simulink model "Furuta_pendulum"  (R2022b)
settings: Solver=ode45  StartTime=0.0  StopTime=3  MaxStep=0.1  RelTol=1e-3
values from neighbouring files (symbols this model uses):
  A = [ 0 0 1 0 ... (first row only)    [Initialize_parameters.m]    (also in Matlab_simulation.m)
  B = [ 0 0 ... (first row only)    [Initialize_parameters.m]    (also in Matlab_simulation.m)
  b1 = 0.01    [Initialize_parameters.m]    (also in Matlab_simulation.m)
  b1s = 0.00    (= 0)    [Initialize_parameters.m]    (also in Matlab_simulation.m = 0.001)
  b2 = 0.001    [Initialize_parameters.m]    (also in Matlab_simulation.m)
  C = ident    [Initialize_parameters.m]    (also in sysCLode.m = [ m2*l2^2*dth2*sin(th2)*cos(th2)+b1,          m2*l2^2*dth1*s)
  D = zeros(4,2)    [Initialize_parameters.m]
  epsilon = 1/sqrt(2)    [Initialize_parameters.m]
  g = 9.81    [Initialize_parameters.m]    (also in Matlab_simulation.m)
  ident = eye(4)    [Initialize_parameters.m]
  invC = inv(C)    [Initialize_parameters.m]
  J1 = 0.000027+0.00257    (= 0.002597)    [Initialize_parameters.m]    (also in Matlab_simulation.m)
  J2 = 4.15e-5    (= 4.15e-05)    [Initialize_parameters.m]    (also in Matlab_simulation.m)
  Ki = 2    [Initialize_parameters.m]
  Kt = 0.071    [Initialize_parameters.m]
  l1 = 0.16    [Initialize_parameters.m]    (also in Matlab_simulation.m)
  l2 = 0.075    [Initialize_parameters.m]    (also in Matlab_simulation.m)
  m2 = 0.0206    [Initialize_parameters.m]    (also in Matlab_simulation.m)
  tau2 = 0.00    (= 0)    [Initialize_parameters.m]    (also in sysCLode.m)
  Td = 0.01    [Initialize_parameters.m]
  tr = 3    [Initialize_parameters.m]
  ts_ZH = 0.001    [Initialize_parameters.m]
  Vmax = 3    [Initialize_parameters.m]
  x0 = [0; 5*deg2rad; 0; 0]    [Initialize_parameters.m]    (also in Matlab_simulation.m = [0; 5*pi/180; 0; 0])
  x_eq = [0; 0; 0; 0]    [Initialize_parameters.m]    (also in Matlab_simulation.m)
undefined symbols (not defined in the file or in its folder): Kinf
settings Model: Creator=lucaschenato  LastModifiedBy=luca.salviato
settings SolverCC: AlgebraicLoopSolver=TrustRegion
settings DataIOCC: ReturnWorkspaceOutputs=off
settings DebuggingCC: UnconnectedInputMsg=warning  UnconnectedOutputMsg=warning  UnconnectedLineMsg=warning  SFMachineParentedDataDiag=warning  ArithmeticOperatorsInVariantConditions=warning
settings ModelReferenceCC: EnableRefExpFcnMdlSchedulingChecks=on
settings SFSimCC: CustomCodeUndefinedFunction=UseInterfaceOnly

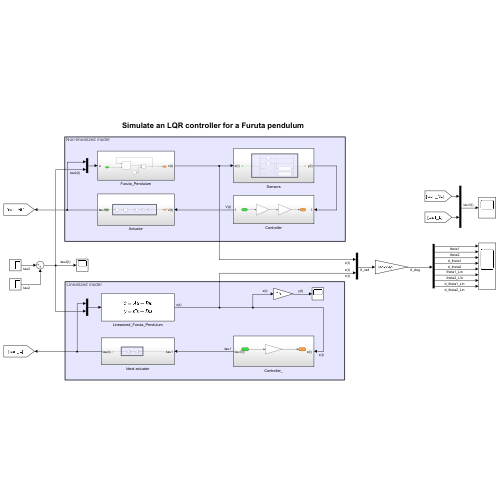
[thumbnail: Simulink's stored preview of the top-level diagram]
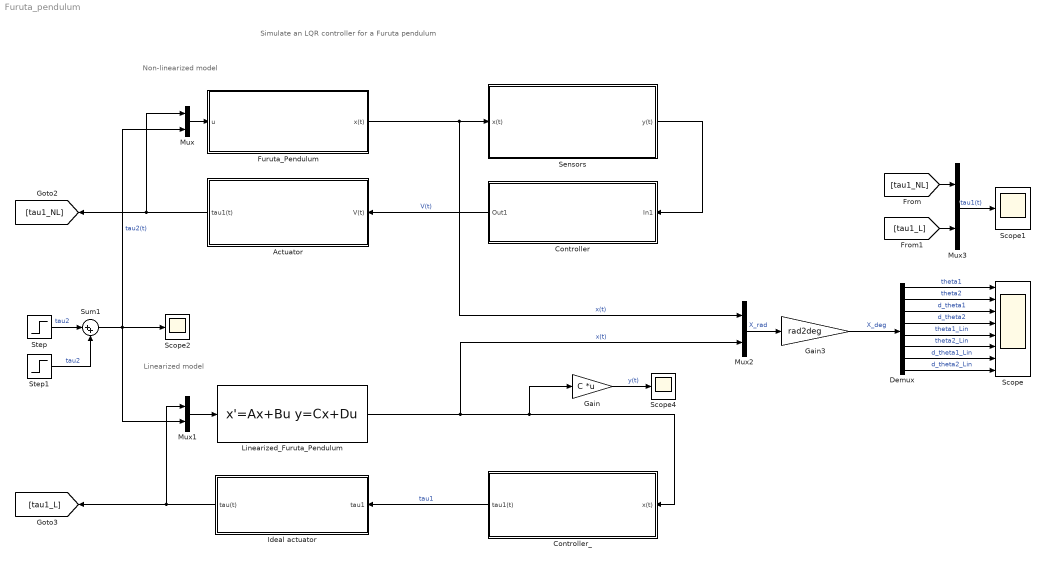
== system Furuta_pendulum ==
  note: Simulate an LQR controller for a Furuta pendulum
  note: Non-linearized model
  note: Linearized model
  Actuator : Subsystem
  Controller : Subsystem
  Controller_ : Subsystem
  Demux : Demux  Outputs=8
  Furuta_Pendulum : Subsystem
  Gain : Gain  Gain=C  Multiplication=Matrix(K*u)
  Gain3 : Gain  Gain=rad2deg
  Ideal actuator : Subsystem
  Linearized_Furuta_Pendulum : StateSpace  A=A  B=B  C=ident  D=D  InitialCondition=x0-x_eq  AbsoluteTolerance=1e-6
  Mux{,1..3} (4 alike) : Mux  Inputs=2
  Scope : Scope  NumInputPorts=8
  Scope1 : Scope
  Scope2 : Scope
  Scope4 : Scope
  Sensors : Subsystem
  Step : Step  Time=tr  After=tau2  SampleTime=0
  Step1 : Step  Time=tr+0.1  After=-tau2  SampleTime=0
  Sum1 : Sum  Inputs=|++
  wires:
  Mux/1 -> Furuta_Pendulum/1(u)
  Linearized_Furuta_Pendulum/1 -> Controller_/1("x(t) "), Gain/1, Mux2/2  "x(t)"
  Mux1/1 -> Linearized_Furuta_Pendulum/1
  Step/1 -> Sum1/1  "tau2"
  Step1/1 -> Sum1/2  "tau2"
  Sum1/1 -> Mux1/2, Mux/2, Scope2/1  "tau2(t)"
  Furuta_Pendulum/1(x(t)) -> Sensors/1(x(t)), Mux2/1  "x(t)"
  Mux2/1 -> Gain3/1  "X_rad"
  Gain/1 -> Scope4/1  "y(t)"
  [tau1_NL] -> Mux3/1
  Mux3/1 -> Scope1/1  "tau1(t)"
  [tau1_L] -> Mux3/2
  Gain3/1 -> Demux/1  "X_deg"
  Demux/1 -> Scope/1  "theta1"
  Demux/2 -> Scope/2  "theta2"
  Demux/3 -> Scope/3  "d_theta1"
  Demux/4 -> Scope/4  "d_theta2"
  Demux/5 -> Scope/5  "theta1_Lin"
  Demux/6 -> Scope/6  "theta2_Lin"
  Demux/7 -> Scope/7  "d_theta1_Lin"
  Demux/8 -> Scope/8  "d_theta2_Lin"
  Sensors/1(y(t)) -> Controller/1(In1)
  Controller/1(Out1) -> Actuator/1(V(t))  "V(t)"
  Actuator/1(tau1(t)) -> [tau1_NL], Mux/1
  Ideal actuator/1(tau(t)) -> Mux1/1, [tau1_L]
  Controller_/1(tau1(t)) -> Ideal actuator/1(tau1)  "tau1"

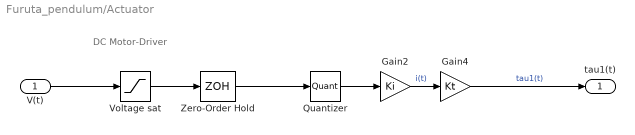
== system Furuta_pendulum/Actuator ==
  note: DC Motor-Driver
  V(t) : Inport
  Gain2 : Gain  Gain=Ki
  Gain4 : Gain  Gain=Kt
  Quantizer : Quantizer  QuantizationInterval=q_DAC
  Voltage sat : Saturate  UpperLimit=Vmax  LowerLimit=-Vmax
  Zero-Order Hold : ZeroOrderHold  SampleTime=ts_ZH
  tau1(t) : Outport
  wires:
  Gain2/1 -> Gain4/1  "i(t)"
  Voltage sat/1 -> Zero-Order Hold/1
  Quantizer/1 -> Gain2/1
  Zero-Order Hold/1 -> Quantizer/1
  Gain4/1 -> tau1(t)/1  "tau1(t)"
  V(t)/1 -> Voltage sat/1

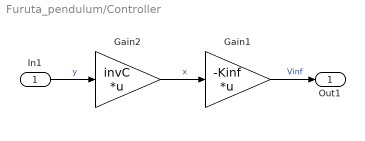
== system Furuta_pendulum/Controller ==
  In1 : Inport
  Gain1 : Gain  Gain=-Kinf  Multiplication=Matrix(K*u)
  Gain2 : Gain  Gain=invC  Multiplication=Matrix(K*u)
  Out1 : Outport
  wires:
  Gain1/1 -> Out1/1  "Vinf"
  In1/1 -> Gain2/1  "y"
  Gain2/1 -> Gain1/1  "x"

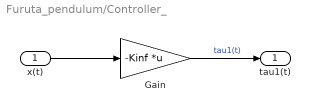
== system Furuta_pendulum/Controller_ ==
  "x(t) " : Inport
  Gain : Gain  Gain=-Kinf  Multiplication=Matrix(K*u)
  tau1(t) : Outport  VectorParamsAs1DForOutWhenUnconnected=off
  wires:
  Gain/1 -> tau1(t)/1  "tau1(t)"
  "x(t) "/1 -> Gain/1

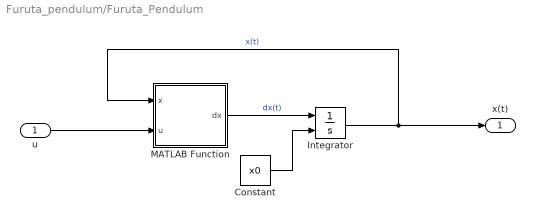
== system Furuta_pendulum/Furuta_Pendulum ==
  u : Inport
  Constant : Constant  Value=x0
  Integrator : Integrator  InitialConditionSource=external  InitialCondition=x0
  MATLAB Function : MATLAB Function  TreatAsAtomicUnit=on
  x(t) : Outport  VectorParamsAs1DForOutWhenUnconnected=off
  wires:
  u/1 -> MATLAB Function/2(u)
  Constant/1 -> Integrator/2
  MATLAB Function/1(dx) -> Integrator/1  "dx(t)"
  Integrator/1 -> x(t)/1, MATLAB Function/1(x)  "x(t)"

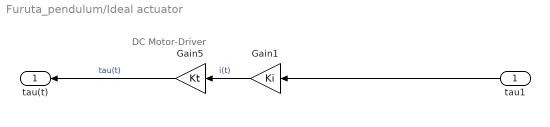
== system Furuta_pendulum/Ideal actuator ==
  note: DC Motor-Driver
  tau1 : Inport
  Gain1 : Gain  Gain=Ki
  Gain5 : Gain  Gain=Kt
  tau(t) : Outport
  wires:
  Gain5/1 -> tau(t)/1  "tau(t)"
  Gain1/1 -> Gain5/1  "i(t)"
  tau1/1 -> Gain1/1

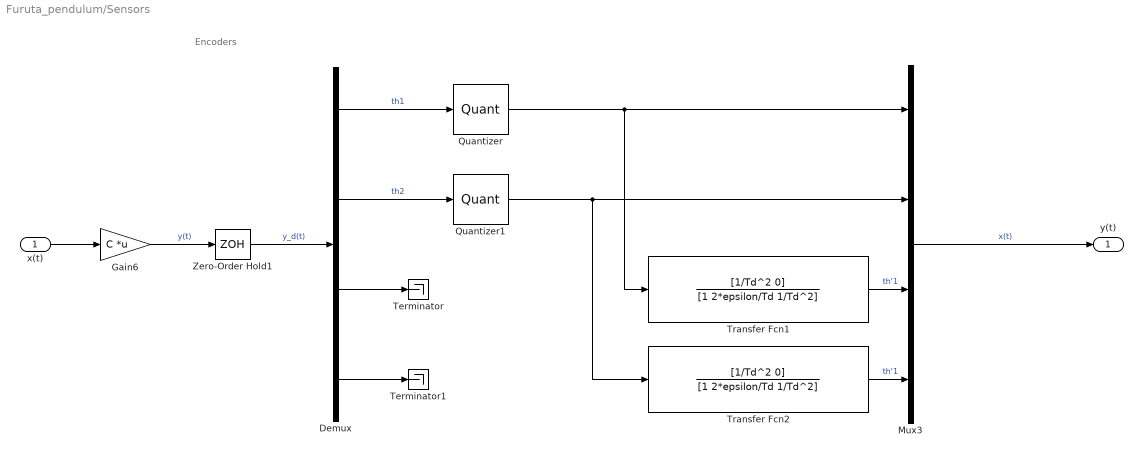
== system Furuta_pendulum/Sensors ==
  note: Encoders
  x(t) : Inport
  Demux : Demux
  Gain6 : Gain  Gain=C  Multiplication=Matrix(K*u)
  Mux3 : Mux
  Quantizer : Quantizer  QuantizationInterval=encoder_res
  Quantizer1 : Quantizer  QuantizationInterval=encoder_res
  Terminator : Terminator
  Terminator1 : Terminator
  Transfer Fcn1 : TransferFcn  Numerator=[1/Td^2 0]  Denominator=[1 2*epsilon/Td 1/Td^2]
  Transfer Fcn2 : TransferFcn  Numerator=[1/Td^2 0]  Denominator=[1 2*epsilon/Td 1/Td^2]
  Zero-Order Hold1 : ZeroOrderHold  SampleTime=ts_ZH
  y(t) : Outport
  wires:
  Zero-Order Hold1/1 -> Demux/1  "y_d(t)"
  Gain6/1 -> Zero-Order Hold1/1  "y(t)"
  x(t)/1 -> Gain6/1
  Quantizer1/1 -> Transfer Fcn2/1, Mux3/2
  Quantizer/1 -> Transfer Fcn1/1, Mux3/1
  Transfer Fcn2/1 -> Mux3/4  "th'1"
  Mux3/1 -> y(t)/1  "x(t)"
  Demux/1 -> Quantizer/1  "th1"
  Demux/2 -> Quantizer1/1  "th2"
  Demux/3 -> Terminator/1
  Transfer Fcn1/1 -> Mux3/3  "th'1"
  Demux/4 -> Terminator1/1

== matlab function Furuta_pendulum/Furuta_Pendulum/MATLAB Function ==
  data: x input; u input; dx output; J1 parameter; J2 parameter; m2 parameter; l1 parameter; l2 parameter; g parameter; b1 parameter; b2 parameter; b1s parameter
function dx = Furuta(x, u, J1, J2, m2, l1, l2, g, b1, b2, b1s)
% FurPar contiene parametri meccanici del Pendolo di 
% Furuta x = [ th1 th2 dth1 dth2]' angoli e loro derivate th1 (rod) e th2 (pendulum) in [rad] e[rad/s] 
% u:  ingressi al sistema u(1) ingresso di controllo u(2) disturbo esterno in [N]
% esterno

th1 = x(1); th2 = x(2);
dth1 = x(3); dth2 = x(4);

% Define nonlinear model: M*ddq + C*dq + G = u
M = [J1+m2*l1^2+m2*l2^2*sin(th2)^2, -m2*l1*l2*cos(th2);
        -m2*l1*l2*cos(th2),          J2 + m2*l2^2 ];

C = [m2*l2^2*dth2*sin(th2)*cos(th2)+b1, m2*l2^2*dth1*sin(th2)*cos(th2)+m2*l1*l2*dth2*sin(th2);
     -m2*l2^2*dth1*sin(th2)*cos(th2),                  b2                                 ];
    
G = [0; -m2*l2*g*sin(th2)];

h = [-b1s*sign(dth1) ; 0];

% Update derivatives
dq = [dth1; dth2];
ddq = M\(-C*dq-G+u+h);
dx = [dq; ddq];
end
